simulink model "Leds"  (R2023b)
settings: Solver=VariableStepAuto  StartTime=0.0  StopTime=10.0  RelTol=1e-3
libraries: simulink x4, arduinolib x3
settings Model: Creator=marqu  LastModifiedBy=marqu

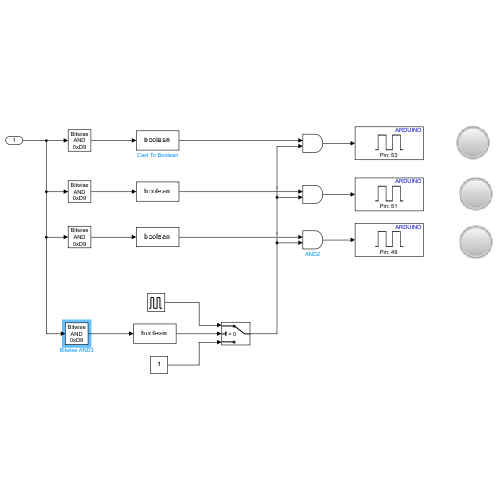
[thumbnail: Simulink's stored preview of the top-level diagram]
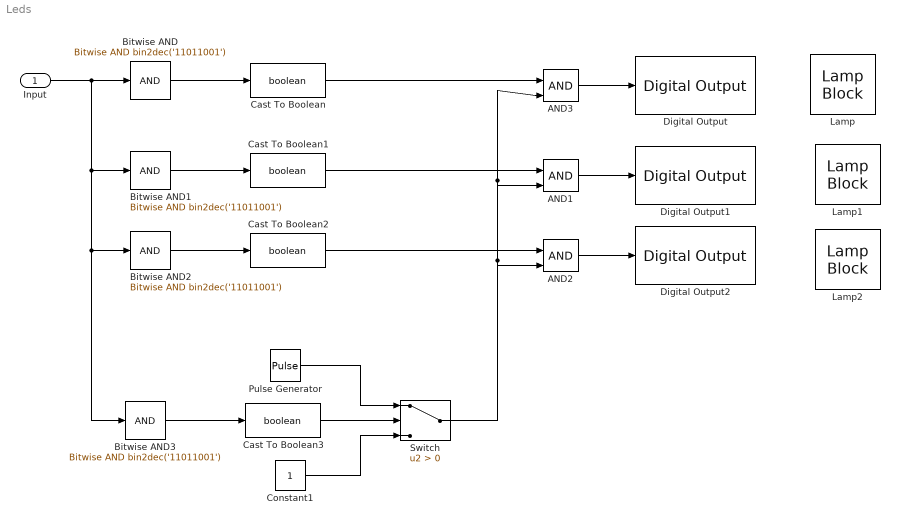
== system Leds ==
  Input : Inport
  AND1 : Logic  IconShape=distinctive  AllPortsSameDT=off  OutDataTypeStr=boolean
  AND2 : Logic  IconShape=distinctive  AllPortsSameDT=off  OutDataTypeStr=boolean
  AND3 : Logic  IconShape=distinctive  AllPortsSameDT=off  OutDataTypeStr=boolean
  Bitwise AND{,1..3} (4 alike) : simulink/Logic and Bit Operations/Bitwise Operator  logicop=AND  UseBitMask=on  BitMask=bin2dec('11011001')  BitMaskRealWorld=Stored Integer
      settings: LibrarySourceBlock=|
      | simulink/Quick Insert/Logic and Bit
      | Operations/Bitwise AND
  Cast To Boolean{,1..3} (4 alike) : DataTypeConversion  OutDataTypeStr=boolean  SaturateOnIntegerOverflow=off  RndMeth=Floor
  Constant1 : Constant
  Digital Output : arduinolib/Digital Output  pinNumber=53  Direction=output  blockPlatform=arduino
  Digital Output1 : arduinolib/Digital Output  pinNumber=51  Direction=output  blockPlatform=arduino
  Digital Output2 : arduinolib/Digital Output  pinNumber=49  Direction=output  blockPlatform=arduino
  Lamp : LampBlock  LabelPosition=Hide
  Lamp1 : LampBlock  LabelPosition=Hide
  Lamp2 : LampBlock  LabelPosition=Hide
  Pulse Generator : DiscretePulseGenerator  PulseType=Time based  Period=10  PulseWidth=5
  Switch : Switch  Criteria=u2 > Threshold  SaturateOnIntegerOverflow=off  InputSameDT=off
  wires:
  Input/1 -> Bitwise AND3/1, Bitwise AND2/1, Bitwise AND1/1, Bitwise AND/1
  Bitwise AND/1 -> Cast To Boolean/1
  Bitwise AND1/1 -> Cast To Boolean1/1
  Bitwise AND2/1 -> Cast To Boolean2/1
  Bitwise AND3/1 -> Cast To Boolean3/1
  Cast To Boolean3/1 -> Switch/2
  Constant1/1 -> Switch/3
  Pulse Generator/1 -> Switch/1
  Switch/1 -> AND2/2, AND1/2, AND3/2
  Cast To Boolean2/1 -> AND2/1
  Cast To Boolean1/1 -> AND1/1
  Cast To Boolean/1 -> AND3/1
  AND3/1 -> Digital Output/1
  AND1/1 -> Digital Output1/1
  AND2/1 -> Digital Output2/1
